simulink model "QianKui"  (R2025b)
settings: Solver=ode4  StartTime=0.0  StopTime=10.0  FixedStep=0.001  RelTol=1e-3
undefined symbols (not defined in the file): LP, SV
settings Model: Creator=J  LastModifiedBy=J

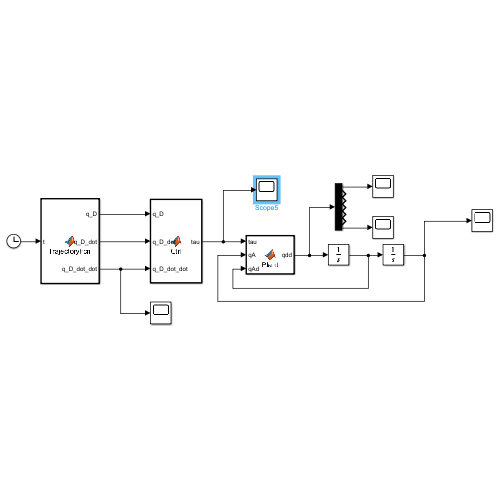
[thumbnail: Simulink's stored preview of the top-level diagram]
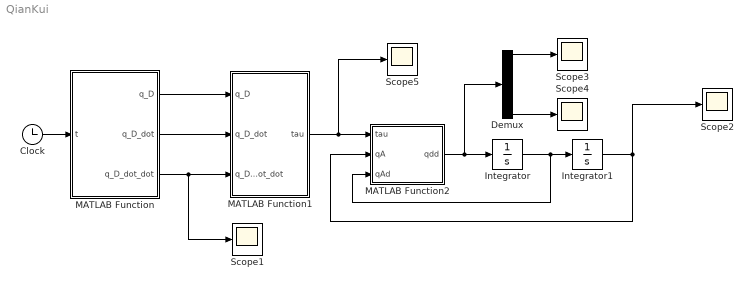
== system QianKui ==
  Clock : Clock
  Demux : Demux  Outputs=7
  Integrator : Integrator
  Integrator1 : Integrator
  MATLAB Function : MATLAB Function  TreatAsAtomicUnit=on
  MATLAB Function1 : MATLAB Function  TreatAsAtomicUnit=on
  MATLAB Function2 : MATLAB Function  TreatAsAtomicUnit=on
  Scope{1..5} (5 alike) : Scope
      Scope1 settings: ActiveDisplayYMinimum=-1  ActiveDisplayYMaximum=1
      Scope2 settings: ActiveDisplayYMinimum=-0.30436158573126104  ActiveDisplayYMaximum=0.58075257988254858  DataLoggingVariableName=ScopeData2
      Scope3 settings: ActiveDisplayYMinimum=-594.87999634836819  ActiveDisplayYMaximum=1697.176088699913
      Scope4 settings: ActiveDisplayYMinimum=-1272.4357390051473  ActiveDisplayYMaximum=3492.5842449930242  DataLoggingVariableName=ScopeData3
      Scope5 settings: ActiveDisplayYMinimum=-30.472382444510789  ActiveDisplayYMaximum=27.328119152358926  DataLoggingVariableName=ScopeData4
  wires:
  Clock/1 -> MATLAB Function/1(t)
  MATLAB Function/1(q_D) -> MATLAB Function1/1(q_D)
  MATLAB Function/2(q_D_dot) -> MATLAB Function1/2(q_D_dot)
  MATLAB Function/3(q_D_dot_dot) -> Scope1/1, MATLAB Function1/3(q_D_dot_dot)
  MATLAB Function1/1(tau) -> Scope5/1, MATLAB Function2/1(tau)
  MATLAB Function2/1(qdd) -> Demux/1, Integrator/1
  Integrator/1 -> MATLAB Function2/3(qAd), Integrator1/1
  Integrator1/1 -> Scope2/1, MATLAB Function2/2(qA)
  Demux/1 -> Scope3/1
  Demux/7 -> Scope4/1

== matlab function QianKui/MATLAB Function1 ==
  data: q_D input size=[7 1]; tau output size=[7 1]; q_D_dot input size=[7 1]; q_D_dot_dot input size=[7 1]; LP parameter; SV parameter
function tau = Ctrl(q_D, q_D_dot, q_D_dot_dot, LP, SV)

q_D = q_D(:);
q_D_dot = q_D_dot(:);
q_D_dot_dot = q_D_dot_dot(:);

[M, C, G] = calc_MCG_0625(LP, SV, q_D, q_D_dot);

tau = M * q_D_dot_dot + C + G;

end

== matlab function QianKui/MATLAB Function ==
  data: t input; q_D output size=[7 1]; q_D_dot output size=[7 1]; q_D_dot_dot output size=[7 1]
function [q_D, q_D_dot, q_D_dot_dot] = TrajectoryFcn(t)

T  = 10;          % 轨迹时间
q0 = [ ...
    0;
    0;
    0;
    0;
    0;
    0;
    0];

qf = [ ...
    0.5;
    0.8;
    1.0;
    0.6;
    1.2;
    0.9;
    0.7];

q_D         = zeros(7,1);
q_D_dot     = zeros(7,1);
q_D_dot_dot = zeros(7,1);

for i = 1:7
    [q_D(i), q_D_dot(i), q_D_dot_dot(i)] = ...
        quintic_traj_0625(t, q0(i), qf(i), T);
end

end

== matlab function QianKui/MATLAB Function2 ==
  data: tau input size=[7 1]; qdd output size=[7 1]; qA input size=[7 1]; qAd input size=[7 1]; LP parameter; SV parameter
function qdd = Plant(tau, qA, qAd, LP, SV)

DIST = 1;

tau = tau(:);
qA  = qA(:);
qAd = qAd(:);

[M, C, G] = calc_MCG_0625(LP, SV, qA, qAd);

qdd = zeros(7,1);

qdd(:) = (DIST * M) \ (tau - DIST * C(:) - DIST * G(:));

end
